simulink model "DC_Motor_OpenLoop"  (R2025b)
settings: Solver=VariableStepAuto  StartTime=0.0  StopTime=10.0  RelTol=1e-3
settings Model: Creator=parminder  LastModifiedBy=parminder

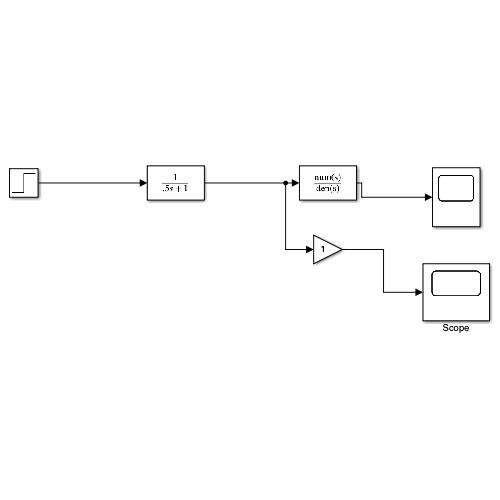
[thumbnail: Simulink's stored preview of the top-level diagram]
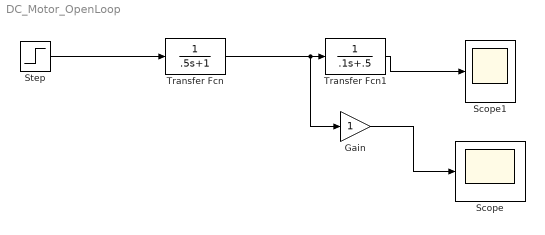
== system DC_Motor_OpenLoop ==
  Gain : Gain
  Scope : Scope
      settings: ActiveDisplayYMinimum=-3.6731333158289639  ActiveDisplayYMaximum=34.773306673436807
  Scope1 : Scope
      settings: ActiveDisplayYMinimum=-232.96241452484747  ActiveDisplayYMaximum=222.81571851337773
  Step : Step  Time=0  After=12  SampleTime=0
  Transfer Fcn : TransferFcn  Denominator=[.5 1]
  Transfer Fcn1 : TransferFcn  Denominator=[.1 .5]
  wires:
  Step/1 -> Transfer Fcn/1
  Transfer Fcn/1 -> Gain/1, Transfer Fcn1/1
  Transfer Fcn1/1 -> Scope1/1
  Gain/1 -> Scope/1
